simulink model "RelayFeedback"  (R2018a)
settings: Solver=VariableStepAuto  StartTime=0.0  StopTime=50.0  RelTol=1e-3
settings Model: Creator=xiangyuliu  LastModifiedBy=xiangyuliu

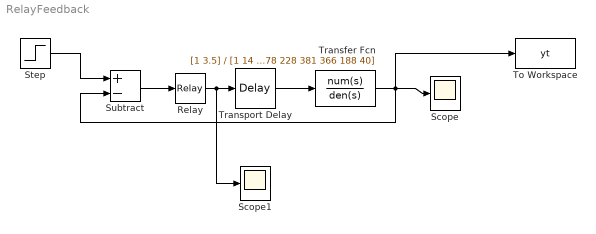
== system RelayFeedback ==
  Relay : Relay  OnSwitchValue=1  OffSwitchValue=1  OffOutputValue=-1
  Scope : Scope
  Scope1 : Scope
  Step : Step  Time=0  SampleTime=0
  Subtract : Sum  Inputs=+-
  To Workspace : ToWorkspace  VariableName=yt  SaveFormat=Timeseries  SampleTime=-1
  Transfer Fcn : TransferFcn  Numerator=[1 3.5]  Denominator=[1 14 78 228 381 366 188 40]
  Transport Delay : TransportDelay  DelayTime=2.5
  wires:
  Subtract/1 -> Relay/1
  Step/1 -> Subtract/1
  Relay/1 -> Scope1/1, Transport Delay/1
  Transfer Fcn/1 -> To Workspace/1, Subtract/2, Scope/1
  Transport Delay/1 -> Transfer Fcn/1
